simulink library "sft"  (Simulink 8.1)
settings: Solver=ode1  StartTime=0.0  StopTime=Inf  FixedStep=0.001  RelTol=1e-3
PostLoadFcn:
  | , if any(exist('dsrtsu_mdlpostloadfcn', 'file') == [2, 3, 6]), try dsrtsu_mdlpostloadfcn('Execute', bdroot); catch fprintf('Error in PostLoadFcn (dsrtsu_mdlpostloadfcn) for model "%s":\n %s\n', bdroot, lasterr); end, end,
libraries: dsf x1, vst x1
settings Model: DSRTSU_INTERNAL_RTI_VER=450  DSRTSU_INTERNAL_RTI_TYPE=rti1401  RTICANMMDATA=struct('GeneralSetupData',struct('modelroot','D:\ELN150201_TAIWAN\trunk\AdasDragon\software\sw_development\arch\app\ifo','generalsettings',struct('filesettings',struct('destfolder',struct('Name','RTICANMM_FILES','Check',1),'buildfolder',struct('Name','.','Check',1),'AbsDestfolder',struct('Name','D:\ELN150201_TAIWAN\trunk\AdasDragon\software\sw_development\arch\app\ifo\RTICANMM_FILES'),'AbsBuildfolder',struct('Name','D:\ELN150201_TAIWAN\trunk\AdasDragon\software\sw_development\arch\app\ifo'))),'options',struct('addpaths',1,'rmpaths',1,'addtrcexclusion',logical(1),'cannavigator',struct('checkmonitoring',0),'show_usrtrc',0,'use_usrtrc',0),'advanced',struct('options',[1 1 1 1 1 1 1 1 1 1 1 1 1 1 1 1 1 1 1 1 1 1 1 1 1 1 1 1 1 1 1 1 1 1 1 1 1 1 1 1 1 1 1 1 1 1 1 1 1 1 1 1 1 1 1 1 1 1 1 1 1 1 1 1 1 1 1 1 1 1 1 1 1 1 1 1 1 1 1 1 1 1 1 1 1 1 1 1 1 1 1 1 1 1 1 1 1 1 1 1]),'MPSetup',{{}},'modelname','sft','block','sft'))  DSRTSU_INTERNAL_RTIFPGA=40  Creator=AT015411  LastModifiedBy=AT015555

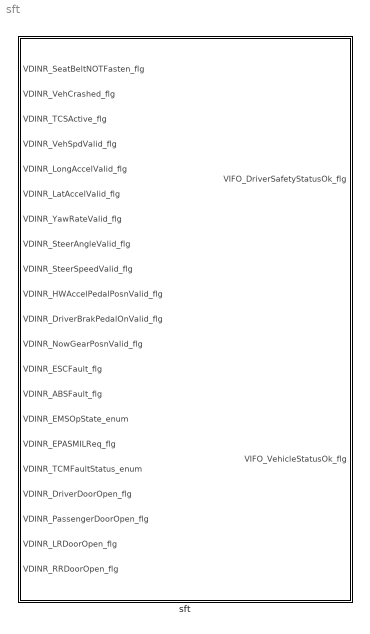
== system sft ==
  sft : Subsystem

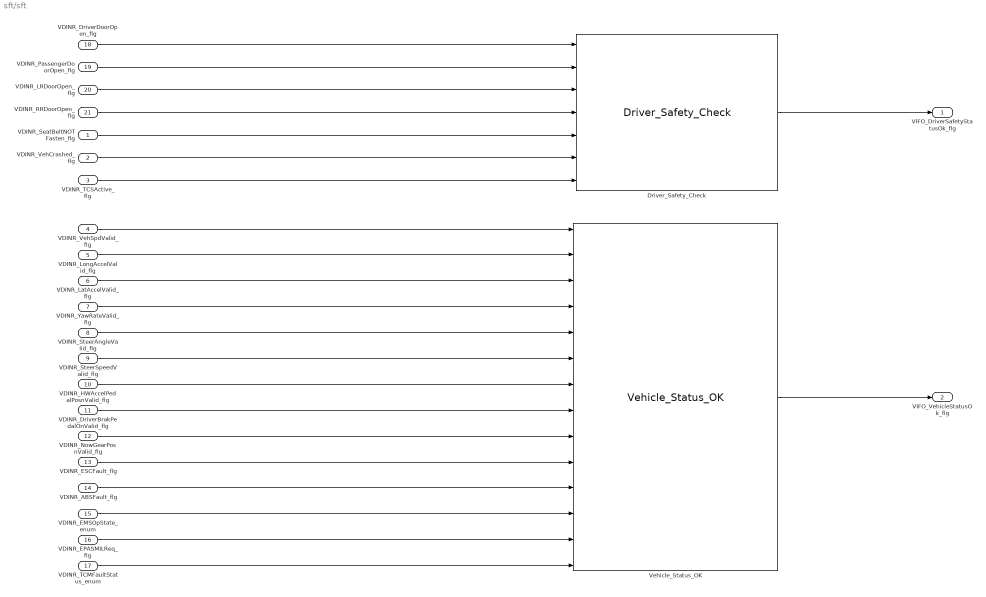
== system sft/sft ==
  VDINR_SeatBeltNOTFasten_flg : Inport
  VDINR_VehCrashed_flg : Inport  Port=2
  VDINR_TCSActive_flg : Inport  Port=3
  VDINR_VehSpdValid_flg : Inport  Port=4
  VDINR_LongAccelValid_flg : Inport  Port=5
  VDINR_LatAccelValid_flg : Inport  Port=6
  VDINR_YawRateValid_flg : Inport  Port=7
  VDINR_SteerAngleValid_flg : Inport  Port=8
  VDINR_SteerSpeedValid_flg : Inport  Port=9
  VDINR_HWAccelPedalPosnValid_flg : Inport  Port=10
  VDINR_DriverBrakPedalOnValid_flg : Inport  Port=11
  VDINR_NowGearPosnValid_flg : Inport  Port=12
  VDINR_ESCFault_flg : Inport  Port=13
  VDINR_ABSFault_flg : Inport  Port=14
  VDINR_EMSOpState_enum : Inport  Port=15
  VDINR_EPASMILReq_flg : Inport  Port=16
  VDINR_TCMFaultStatus_enum : Inport  Port=17
  VDINR_DriverDoorOpen_flg : Inport  Port=18
  VDINR_PassengerDoorOpen_flg : Inport  Port=19
  VDINR_LRDoorOpen_flg : Inport  Port=20
  VDINR_RRDoorOpen_flg : Inport  Port=21
  Driver_Safety_Check : dsf/Driver_Safety_Check
  Vehicle_Status_OK : vst/Vehicle_Status_OK
  VIFO_DriverSafetyStatusOk_flg : Outport
  VIFO_VehicleStatusOk_flg : Outport  Port=2
  wires:
  VDINR_DriverDoorOpen_flg/1 -> Driver_Safety_Check/1
  VDINR_PassengerDoorOpen_flg/1 -> Driver_Safety_Check/2
  VDINR_LRDoorOpen_flg/1 -> Driver_Safety_Check/3
  VDINR_RRDoorOpen_flg/1 -> Driver_Safety_Check/4
  VDINR_SeatBeltNOTFasten_flg/1 -> Driver_Safety_Check/5
  VDINR_VehCrashed_flg/1 -> Driver_Safety_Check/6
  VDINR_TCSActive_flg/1 -> Driver_Safety_Check/7
  Vehicle_Status_OK/1 -> VIFO_VehicleStatusOk_flg/1
  VDINR_TCMFaultStatus_enum/1 -> Vehicle_Status_OK/14
  VDINR_EPASMILReq_flg/1 -> Vehicle_Status_OK/13
  VDINR_EMSOpState_enum/1 -> Vehicle_Status_OK/12
  VDINR_ABSFault_flg/1 -> Vehicle_Status_OK/11
  VDINR_ESCFault_flg/1 -> Vehicle_Status_OK/10
  VDINR_NowGearPosnValid_flg/1 -> Vehicle_Status_OK/9
  VDINR_DriverBrakPedalOnValid_flg/1 -> Vehicle_Status_OK/8
  VDINR_HWAccelPedalPosnValid_flg/1 -> Vehicle_Status_OK/7
  VDINR_SteerSpeedValid_flg/1 -> Vehicle_Status_OK/6
  VDINR_SteerAngleValid_flg/1 -> Vehicle_Status_OK/5
  VDINR_YawRateValid_flg/1 -> Vehicle_Status_OK/4
  VDINR_VehSpdValid_flg/1 -> Vehicle_Status_OK/1
  VDINR_LatAccelValid_flg/1 -> Vehicle_Status_OK/3
  VDINR_LongAccelValid_flg/1 -> Vehicle_Status_OK/2
  Driver_Safety_Check/1 -> VIFO_DriverSafetyStatusOk_flg/1
